simulink model "quadsim_ver2011b"  (Simulink 7.8)
settings: Solver=ode23  StartTime=0.0  StopTime=140  RelTol=1e-3
undefined symbols (not defined in the file): P, quadsim_control, quadsim_display, quadsim_estimates, quadsim_forces_moments, quadsim_kin_dyn, quadsim_logging, quadsim_sensors, quadsim_truth_feedback, quadsim_wind
libraries: simulink x9
settings Model: Creator=bartojd1  LastModifiedBy=bartojd1
settings DataIOCC: SaveOutput=off  SignalLogging=off  SaveTime=off
settings DebuggingCC: UnderspecifiedInitializationDetection=Simplified  MergeDetectMultiDrivingBlocksExec=error  FcnCallInpInsideContextMsg=Use local settings
settings CodeAppCC: CustomSymbolStrType=$N$R$M_T
settings GRTTargetCC: TargetFunctionLibrary=C89/C90 (ANSI)

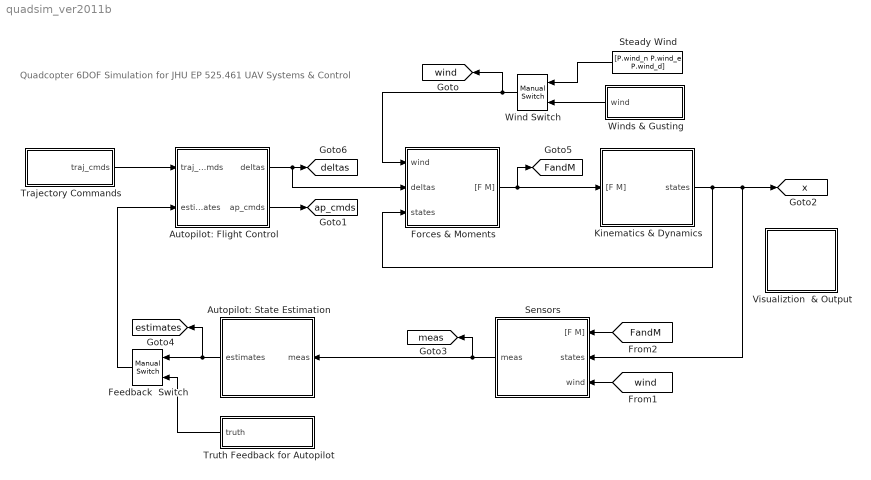
== system quadsim_ver2011b ==
  note: Quadcopter 6DOF Simulation
      | for JHU EP 525.461
      | UAV Systems & Control
  Autopilot: Flight Control : Subsystem
  Autopilot: State Estimation : Subsystem
  Feedback  Switch : simulink/Signal Routing/Manual Switch  sw=0  action=0  varsize=off
  Forces & Moments : Subsystem
  Kinematics & Dynamics : Subsystem
  Sensors : Subsystem
  Steady Wind : Constant  Value=[P.wind_n P.wind_e P.wind_d]
  Trajectory Commands : Subsystem
  Truth Feedback for Autopilot : Subsystem
  Visualiztion  & Output : Subsystem
  Wind Switch : simulink/Signal Routing/Manual Switch  sw=1  action=0  varsize=off
  Winds & Gusting : Subsystem
  tag scope: FandM=global, ap_cmds=global, deltas=global, estimates=global, meas=global, wind=global, x=global
  wires:
  Kinematics & Dynamics/1(states) -> Forces & Moments/3(states), [x], Sensors/2(states)
  Forces & Moments/1("[F M]") -> Kinematics & Dynamics/1("[F M]"), [FandM]
  Sensors/1(meas) -> Autopilot: State Estimation/1(meas), [meas]
  [wind] -> Sensors/3(wind)
  Autopilot: Flight Control/2(ap_cmds) -> [ap_cmds]
  [FandM] -> Sensors/1("[F M]")
  Trajectory Commands/1(" traj_cmds") -> Autopilot: Flight Control/1(traj_cmds)
  Winds & Gusting/1(wind) -> Wind Switch/2
  Wind Switch/1 -> Forces & Moments/1("wind  "), [wind]
  Steady Wind/1 -> Wind Switch/1
  Autopilot: Flight Control/1(deltas) -> [deltas], Forces & Moments/2(deltas)
  Autopilot: State Estimation/1(estimates) -> Feedback  Switch/1, [estimates]
  Feedback  Switch/1 -> Autopilot: Flight Control/2(estimates)
  Truth Feedback for Autopilot/1(truth) -> Feedback  Switch/2

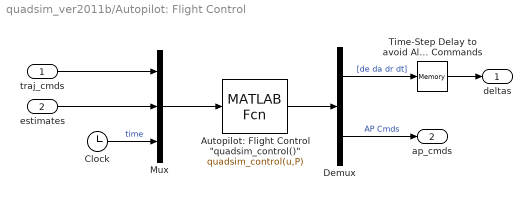
== system quadsim_ver2011b/Autopilot: Flight Control ==
  traj_cmds : Inport
  estimates : Inport  Port=2
  "Autopilot: Flight Control \"quadsim_control()\"" : MATLABFcn  MATLABFcn=quadsim_control(u,P)  OutputDimensions=4+9  SampleTime="P.Ts     % Autopilot at 100Hz"
  Clock : Clock
  Demux : Demux  Outputs=[4;9]
  Mux : Mux  Inputs=3
  Time-Step Delay to avoid Algepraic Loop I.C.: Trim Commands : Memory  X0=[P.delta_e0 P.delta_a0 P.delta_r0 P.delta_t0]'
  deltas : Outport
  ap_cmds : Outport  Port=2
  wires:
  Clock/1 -> Mux/3  "time"
  "Autopilot: Flight Control \"quadsim_control()\""/1 -> Demux/1
  Mux/1 -> "Autopilot: Flight Control \"quadsim_control()\""/1
  estimates/1 -> Mux/2
  traj_cmds/1 -> Mux/1
  Demux/2 -> ap_cmds/1  "AP Cmds"
  Demux/1 -> Time-Step Delay to avoid Algepraic Loop I.C.: Trim Commands/1  "[de da dr dt]"
  Time-Step Delay to avoid Algepraic Loop I.C.: Trim Commands/1 -> deltas/1

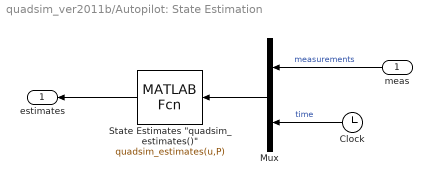
== system quadsim_ver2011b/Autopilot: State Estimation ==
  meas : Inport
  Clock : Clock
  Mux : Mux  Inputs=2
  "State Estimates \"quadsim_estimates()\"" : MATLABFcn  MATLABFcn=quadsim_estimates(u,P)  OutputDimensions=23  SampleTime="P.Ts   % Autopilot at 100 Hz"
  estimates : Outport
  wires:
  meas/1 -> Mux/1  "measurements"
  Mux/1 -> "State Estimates \"quadsim_estimates()\""/1
  Clock/1 -> Mux/2  "time"
  "State Estimates \"quadsim_estimates()\""/1 -> estimates/1

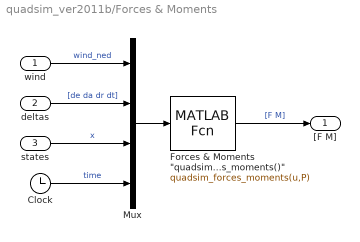
== system quadsim_ver2011b/Forces & Moments ==
  "wind  " : Inport
  deltas : Inport  Port=2
  states : Inport  Port=3
  Clock : Clock
  "Forces & Moments \"quadsim_forces_moments()\"" : MATLABFcn  MATLABFcn=quadsim_forces_moments(u,P)  OutputDimensions=3+3 % (3 forces), (3 moments)
  Mux : Mux
  "[F M]" : Outport
  wires:
  "Forces & Moments \"quadsim_forces_moments()\""/1 -> "[F M]"/1  "[F M]"
  Mux/1 -> "Forces & Moments \"quadsim_forces_moments()\""/1
  Clock/1 -> Mux/4  "time"
  "wind  "/1 -> Mux/1  "wind_ned"
  deltas/1 -> Mux/2  "[de da dr dt]"
  states/1 -> Mux/3  "x"

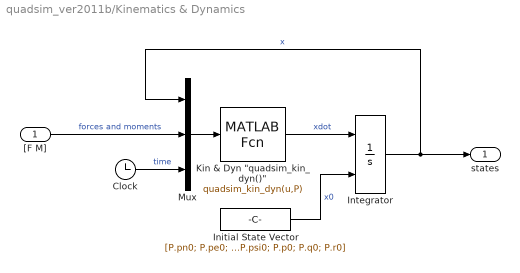
== system quadsim_ver2011b/Kinematics & Dynamics ==
  "[F M]" : Inport
  Clock : Clock
  Initial State Vector : Constant  Value=[P.pn0; P.pe0; P.pd0; P.u0; P.v0; P.w0; P.phi0; P.theta0; P.psi0; P.p0; P.q0; P.r0]
  Integrator : Integrator  InitialConditionSource=external
  "Kin & Dyn \"quadsim_kin_dyn()\"" : MATLABFcn  MATLABFcn=quadsim_kin_dyn(u,P)  OutputDimensions=12
  Mux : Mux  Inputs=3
  states : Outport
  wires:
  Integrator/1 -> Mux/1, states/1  "x"
  Mux/1 -> "Kin & Dyn \"quadsim_kin_dyn()\""/1
  "Kin & Dyn \"quadsim_kin_dyn()\""/1 -> Integrator/1  "xdot"
  "[F M]"/1 -> Mux/2  "forces and moments"
  Initial State Vector/1 -> Integrator/2  "x0"
  Clock/1 -> Mux/3  "time"

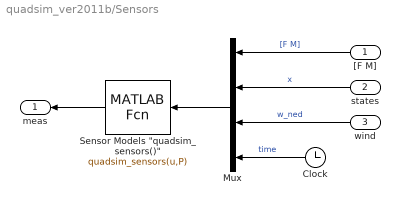
== system quadsim_ver2011b/Sensors ==
  "[F M]" : Inport
  states : Inport  Port=2
  wind : Inport  Port=3
  Clock : Clock
  Mux : Mux
  "Sensor Models \"quadsim_sensors()\"" : MATLABFcn  MATLABFcn=quadsim_sensors(u,P)  OutputDimensions=18
  meas : Outport
  wires:
  Mux/1 -> "Sensor Models \"quadsim_sensors()\""/1
  "Sensor Models \"quadsim_sensors()\""/1 -> meas/1
  Clock/1 -> Mux/4  "time"
  "[F M]"/1 -> Mux/1  "[F M]"
  states/1 -> Mux/2  "x"
  wind/1 -> Mux/3  "w_ned"

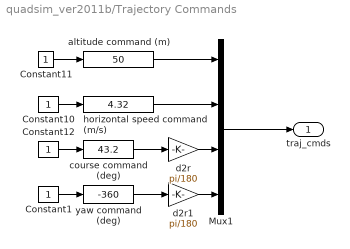
== system quadsim_ver2011b/Trajectory Commands ==
  Constant{1,10..12} (4 alike) : Constant
  Mux1 : Mux
  altitude command (m) : simulink/Math Operations/Slider Gain  low=0  gain=50  high=100
  course command (deg) : simulink/Math Operations/Slider Gain  low=-360  gain=43.2  high=360
  d2r : Gain  Gain=pi/180
  d2r1 : Gain  Gain=pi/180
  horizontal speed command (m/s) : simulink/Math Operations/Slider Gain  low=0  gain=4.32  high=18
  yaw command (deg) : simulink/Math Operations/Slider Gain  low=-360  gain=-360  high=360
  " traj_cmds" : Outport
  wires:
  Constant12/1 -> course command (deg)/1
  course command (deg)/1 -> d2r/1
  d2r/1 -> Mux1/3
  Mux1/1 -> " traj_cmds"/1
  Constant1/1 -> yaw command (deg)/1
  yaw command (deg)/1 -> d2r1/1
  d2r1/1 -> Mux1/4
  Constant10/1 -> horizontal speed command (m/s)/1
  horizontal speed command (m/s)/1 -> Mux1/2
  Constant11/1 -> altitude command (m)/1
  altitude command (m)/1 -> Mux1/1

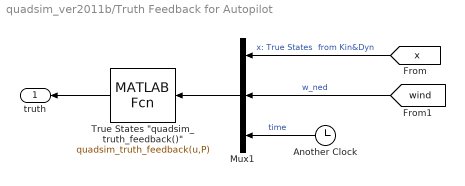
== system quadsim_ver2011b/Truth Feedback for Autopilot ==
  Another Clock : Clock
  Mux1 : Mux  Inputs=3
  "True States \"quadsim_truth_feedback()\"" : MATLABFcn  MATLABFcn=quadsim_truth_feedback(u,P)  OutputDimensions=23  SampleTime="P.Ts   % Autopilot at 100 Hz"
  truth : Outport
  wires:
  Mux1/1 -> "True States \"quadsim_truth_feedback()\""/1
  [x] -> Mux1/1  "x: True States  from Kin&Dyn"
  [wind] -> Mux1/2  "w_ned"
  Another Clock/1 -> Mux1/3  "time"
  "True States \"quadsim_truth_feedback()\""/1 -> truth/1

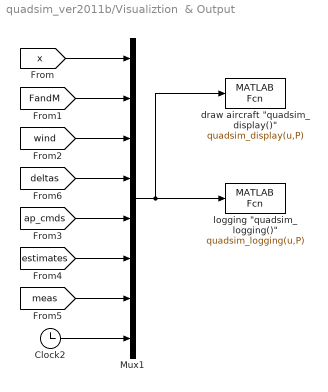
== system quadsim_ver2011b/Visualiztion  & Output ==
  Clock2 : Clock
  Mux1 : Mux  Inputs=8
  "draw aircraft \"quadsim_display()\"" : MATLABFcn  MATLABFcn=quadsim_display(u,P)  OutputDimensions=0  SampleTime=P.Tvis
  "logging \"quadsim_logging()\"" : MATLABFcn  MATLABFcn=quadsim_logging(u,P)  OutputDimensions=0  SampleTime=P.Tlog
  wires:
  [FandM] -> Mux1/2
  [wind] -> Mux1/3
  Mux1/1 -> "logging \"quadsim_logging()\""/1, "draw aircraft \"quadsim_display()\""/1
  [x] -> Mux1/1
  [deltas] -> Mux1/4
  [ap_cmds] -> Mux1/5
  [estimates] -> Mux1/6
  [meas] -> Mux1/7
  Clock2/1 -> Mux1/8

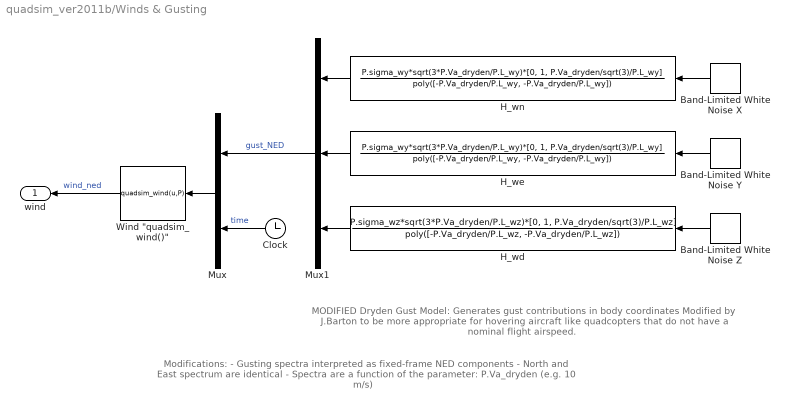
== system quadsim_ver2011b/Winds & Gusting ==
  note: Modifications:
      | - Gusting spectra interpreted as fixed-frame NED components
      | - North and East spectrum are identical
      | - Spectra are a function of the parameter: P.Va_dryden (e.g. 10 m/s)
  note: MODIFIED Dryden Gust Model:
      | Generates gust contributions in body coordinates
      |
      | Modified by J.Barton to be more appropriate for
      | hovering aircraft like quadcopters that do not have
      | a nominal flight airspeed.
  Band-Limited White Noise X : simulink/Sources/Band-Limited White Noise  Cov=[1]  Ts=P.Ts  seed=round(1e9*rand)
  Band-Limited White Noise Y : simulink/Sources/Band-Limited White Noise  Cov=[1]  Ts=P.Ts  seed=round(1e9*rand)
  Band-Limited White Noise Z : simulink/Sources/Band-Limited White Noise  Cov=[1]  Ts=P.Ts  seed=round(1e9*rand)
  Clock : Clock
  H_wd : TransferFcn  Numerator=P.sigma_wz*sqrt(3*P.Va_dryden/P.L_wz)*[0, 1, P.Va_dryden/sqrt(3)/P.L_wz]  Denominator=poly([-P.Va_dryden/P.L_wz, -P.Va_dryden/P.L_wz])
  H_we : TransferFcn  Numerator=P.sigma_wy*sqrt(3*P.Va_dryden/P.L_wy)*[0, 1, P.Va_dryden/sqrt(3)/P.L_wy]  Denominator=poly([-P.Va_dryden/P.L_wy, -P.Va_dryden/P.L_wy])
  H_wn : TransferFcn  Numerator=P.sigma_wy*sqrt(3*P.Va_dryden/P.L_wy)*[0, 1, P.Va_dryden/sqrt(3)/P.L_wy]  Denominator=poly([-P.Va_dryden/P.L_wy, -P.Va_dryden/P.L_wy])
  Mux : Mux  Inputs=2
  Mux1 : Mux  Inputs=3
  "Wind \"quadsim_wind()\"" : MATLABFcn  MATLABFcn=quadsim_wind(u,P)  OutputDimensions=3
  wind : Outport
  wires:
  Mux/1 -> "Wind \"quadsim_wind()\""/1
  "Wind \"quadsim_wind()\""/1 -> wind/1  "wind_ned"
  Clock/1 -> Mux/2  "time"
  Mux1/1 -> Mux/1  "gust_NED"
  H_wn/1 -> Mux1/1
  H_we/1 -> Mux1/2
  H_wd/1 -> Mux1/3
  Band-Limited White Noise X/1 -> H_wn/1
  Band-Limited White Noise Y/1 -> H_we/1
  Band-Limited White Noise Z/1 -> H_wd/1
